simulink model "invertedCinematicDifferential"  (R2018b)
settings: Solver=FixedStepAuto  StartTime=0.0  StopTime=10.0  RelTol=1e-3
values from neighbouring files (symbols this model uses):
  com_des = [x_com,y_com,z_com]    [main.m]
  cond_init = [x1,x2,x3,x4,x5,x6]'    [main.m]
  param = param'    [main.m]
settings Model: Creator=Utente  LastModifiedBy=Utente

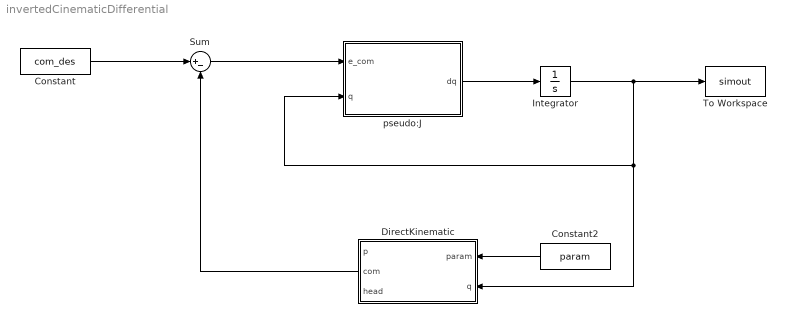
== system invertedCinematicDifferential ==
  Constant : Constant  Value=com_des
  Constant2 : Constant  Value=param
  DirectKinematic : MATLAB Function  TreatAsAtomicUnit=on
  Integrator : Integrator  InitialCondition=cond_init
  Sum : Sum  Inputs=|+-
  To Workspace : ToWorkspace  VariableName=simout  SaveFormat=Timeseries  SampleTime=-1
  pseudo:J : MATLAB Function  TreatAsAtomicUnit=on
  wires:
  Constant/1 -> Sum/1
  Sum/1 -> pseudo:J/1(e_com)
  pseudo:J/1(dq) -> Integrator/1
  Integrator/1 -> To Workspace/1, DirectKinematic/2(q), pseudo:J/2(q)
  DirectKinematic/2(com) -> Sum/2
  Constant2/1 -> DirectKinematic/1(param)

== matlab function invertedCinematicDifferential/DirectKinematic ==
  data: param input; q input; p output; com output; head output
function [p,com,head] = DirectKinematic(param,q)

    x1 = q(1);
    x2 = q(2);
    x3 = q(3);
    x4 = q(4);
    x5 = q(5);
    xhead = q(6);

    a1 = param(1,1);
    a2 = param(2,1);
    a3 = param(3,1);
    a4 = param(4,1);
    a5 = param(5,1);
    a6 = param(6,1);

    m1 = param(1,2);
    m2 = param(2,2);
    m3 = param(3,2);
    m4 = param(4,2);
    m5 = param(5,2);
    m6 = param(6,2);

    angle0_1 = pi/6;
    angle0_2 = 5*pi/6;
    angle0_3 = -3*pi/5;
    angle0_4 = 4*pi/5;
    angle0_5 = pi/10;
    angle0_head = -3*pi/4;

    T1 = matrixDH(a1,0,0,x1);
    T2 = matrixDH(a2,0,0,x2);
    T3 = matrixDH(a3,0,0,x3);
    T4 = matrixDH(a4,0,0,x4);
    T5 = matrixDH(a5,0,0,x5);
    % T6 = matrixDH(a6,0,0,x6+pi/2);

    p0 = [0,0,0]';
    p1 = T1(1:3,4);
    T = T1*T2;
    p2 = T(1:3,4);
    T = T*T3;
    p3 = T(1:3,4);
    T = T*T4;
    p4 = T(1:3,4);
    T = T*T5;
    p5 = T(1:3,4);

    p = [p0,p1,p2,p3,p4,p5]';

    T3_Head = matrixDH(a6,0,0,xhead);
    T_HEAD = T1*T2*T3_Head;
    head = T_HEAD(1:3,4);

    % Com
    C1 = matrixDH(a1/2,0,0,x1);
    C2 = matrixDH(a2/2,0,0,x2);
    C3 = matrixDH(a3/2,0,0,x3);
    C4 = matrixDH(a4/2,0,0,x4);
    C5 = matrixDH(a5/2,0,0,x5);

    %Head
    C_HEAD = matrixDH(a6,0,0,xhead);

    c1 = C1(1:3,4);
    C_m = C1*C2;
    c2 = C_m(1:3,4);
    C_m = C_m*C3;
    c3 = C_m(1:3,4);
    C_m = C_m*C4;
    c4 = C_m(1:3,4);
    C_m = C_m*C5;
    c5 = C_m(1:3,4);

    C_m = C1*C2*C_HEAD;
    c6 = C_m(1:3,4);

    com = (m1*c1 + m2*c2 + m3*c3 + m4*c4 + m5*c5 + m6*c6)...
            / (m1+m2+m3+m4+m5+m6);

end

== matlab function invertedCinematicDifferential/pseudo:J ==
  data: e_com input; dq output; q input
function dq = pseudo_jacobian(e_com,q)
    
    q1 = q(1);
    q2 = q(2);
    q3 = q(3);
    q4 = q(4);
    q5 = q(5);
    q6 = q(6);
    
    K_com = 0.5;
    
    J_com = [ (3*sin(q1 + q2 + q3 + q4 + atan(((5^(1/2) + 5)^(1/2)*(3*2^(1/2) - 10^(1/2)))/4)))/19 - (7*cos(q1 + q2 + q3 - atan(((5 - 5^(1/2))^(1/2)*(5*2^(1/2) - 10^(1/2)))/20)))/38 + (3*cos(q1 + q2 + q3 + q4 + q5 + atan(((2^(1/2) - 10^(1/2))*(5 - 5^(1/2))^(1/2))/4)))/38 + (9*sin(q1 + q2))/19 - (10*sin(q1 + q2 + q6 + pi/4))/19 - sin(q1 + pi/6)/2, (3*sin(q1 + q2 + q3 + q4 + atan(((5^(1/2) + 5)^(1/2)*(3*2^(1/2) - 10^(1/2)))/4)))/19 - (7*cos(q1 + q2 + q3 - atan(((5 - 5^(1/2))^(1/2)*(5*2^(1/2) - 10^(1/2)))/20)))/38 + (3*cos(q1 + q2 + q3 + q4 + q5 + atan(((2^(1/2) - 10^(1/2))*(5 - 5^(1/2))^(1/2))/4)))/38 + (9*sin(q1 + q2))/19 - (10*sin(q1 + q2 + q6 + pi/4))/19, (3*sin(q1 + q2 + q3 + q4 + atan(((5^(1/2) + 5)^(1/2)*(3*2^(1/2) - 10^(1/2)))/4)))/19 - (7*cos(q1 + q2 + q3 - atan(((5 - 5^(1/2))^(1/2)*(5*2^(1/2) - 10^(1/2)))/20)))/38 + (3*cos(q1 + q2 + q3 + q4 + q5 + atan(((2^(1/2) - 10^(1/2))*(5 - 5^(1/2))^(1/2))/4)))/38, (3*sin(q1 + q2 + q3 + q4 + atan(((5^(1/2) + 5)^(1/2)*(3*2^(1/2) - 10^(1/2)))/4)))/19 + (3*cos(q1 + q2 + q3 + q4 + q5 + atan(((2^(1/2) - 10^(1/2))*(5 - 5^(1/2))^(1/2))/4)))/38, (3*cos(q1 + q2 + q3 + q4 + q5 + atan(((2^(1/2) - 10^(1/2))*(5 - 5^(1/2))^(1/2))/4)))/38, -(10*sin(q1 + q2 + q6 + pi/4))/19;
              (3*sin(q1 + q2 + q3 + q4 + q5 + atan(((2^(1/2) - 10^(1/2))*(5 - 5^(1/2))^(1/2))/4)))/38 - (7*sin(q1 + q2 + q3 - atan(((5 - 5^(1/2))^(1/2)*(5*2^(1/2) - 10^(1/2)))/20)))/38 - (9*cos(q1 + q2))/19 - (3*cos(q1 + q2 + q3 + q4 + atan(((5^(1/2) + 5)^(1/2)*(3*2^(1/2) - 10^(1/2)))/4)))/19 + (10*cos(q1 + q2 + q6 + pi/4))/19 + cos(q1 + pi/6)/2, (3*sin(q1 + q2 + q3 + q4 + q5 + atan(((2^(1/2) - 10^(1/2))*(5 - 5^(1/2))^(1/2))/4)))/38 - (7*sin(q1 + q2 + q3 - atan(((5 - 5^(1/2))^(1/2)*(5*2^(1/2) - 10^(1/2)))/20)))/38 - (9*cos(q1 + q2))/19 - (3*cos(q1 + q2 + q3 + q4 + atan(((5^(1/2) + 5)^(1/2)*(3*2^(1/2) - 10^(1/2)))/4)))/19 + (10*cos(q1 + q2 + q6 + pi/4))/19, (3*sin(q1 + q2 + q3 + q4 + q5 + atan(((2^(1/2) - 10^(1/2))*(5 - 5^(1/2))^(1/2))/4)))/38 - (7*sin(q1 + q2 + q3 - atan(((5 - 5^(1/2))^(1/2)*(5*2^(1/2) - 10^(1/2)))/20)))/38 - (3*cos(q1 + q2 + q3 + q4 + atan(((5^(1/2) + 5)^(1/2)*(3*2^(1/2) - 10^(1/2)))/4)))/19, (3*sin(q1 + q2 + q3 + q4 + q5 + atan(((2^(1/2) - 10^(1/2))*(5 - 5^(1/2))^(1/2))/4)))/38 - (3*cos(q1 + q2 + q3 + q4 + atan(((5^(1/2) + 5)^(1/2)*(3*2^(1/2) - 10^(1/2)))/4)))/19, (3*sin(q1 + q2 + q3 + q4 + q5 + atan(((2^(1/2) - 10^(1/2))*(5 - 5^(1/2))^(1/2))/4)))/38,  (10*cos(q1 + q2 + q6 + pi/4))/19;       
                                                                                                                                                                                                                                                                                                                                            0,                                                                                                                                                                                                                                                                                                                          0,                                                                                                                                                                                                                                                                 0,                                                                                                                                                                              0,                                                                                       0,                                 0];
    pinv_J_com = pinv(J_com);

    dq = pinv_J_com*K_com*e_com;

end
